simulink model "LQG"  (R2019a)
settings: Solver=VariableStepAuto  StartTime=0.0  StopTime=50  RelTol=1e-3  EnableMultiTasking=on
values from neighbouring files (symbols this model uses):
  C = [1 0 0 0 0 0]    [FinalProjectENPM667.m]
  K = lqr(A, B, Q, R)    [FinalProjectENPM667.m]
  l1 = 20    [FinalProjectENPM667.m]
  l2 = 10    [FinalProjectENPM667.m]
  M = 1000    [FinalProjectENPM667.m]
  m1 = 100    [FinalProjectENPM667.m]
  m2 = 100    [FinalProjectENPM667.m]
undefined symbols (not defined in the file or in its folder): A1, B1, Continuous, Nbar, Time, X0
libraries: ctrlSharedLib x1
settings Model: Creator=Rishabh  LastModifiedBy=detwieller
settings DataIOCC: ReturnWorkspaceOutputs=off
settings OptimizationCC: LifeSpan=inf
settings DebuggingCC: SFUnexpectedBacktrackingDiag=warning  SFNoUnconditionalDefaultTransitionDiag=warning  SFExecutionAtInitializationDiag=none  ArithmeticOperatorsInVariantConditions=warning
settings SFSimCC: SimUseLocalCustomCode=off
settings RTWCC: RTWUseLocalCustomCode=off
settings CodeAppCC: StateflowObjectComments=on
settings GRTTargetCC: TargetLangStandard=C89/C90 (ANSI)  GeneratePreprocessorConditionals=Disable all
settings ConfigComp: CovMetricSettings=dw  CovHtmlReporting=on  CovSaveCumulativeToWorkspaceVar=on  CovSaveSingleToWorkspaceVar=on  CovExternalEMLEnable=off

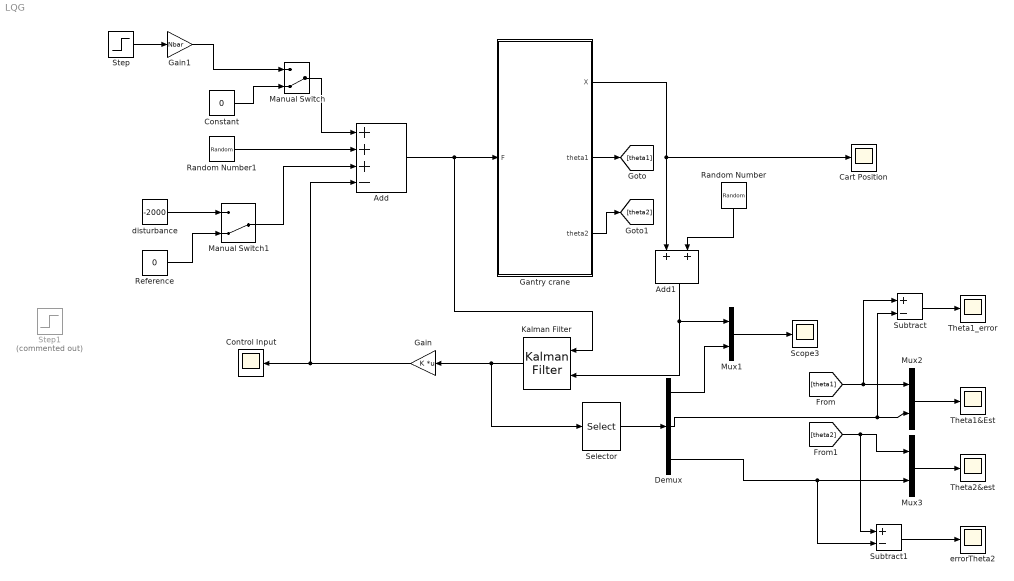
== system LQG ==
  Add : Sum  Inputs=+++-
  Add1 : Sum
  Cart Position : Scope
  Constant : Constant  Value=0
  Control Input : Scope
  Demux : Demux  Outputs=3
  Gain : Gain  Gain=K  Multiplication=Matrix(K*u)
  Gain1 : Gain  Gain=Nbar
  "Gantry crane " : Subsystem
  Kalman Filter : ctrlSharedLib/Kalman Filter  TimeDomain=Continuous-Time  UseCurrentEstimator=on  ModelSource=Individual A, B, C, D matrices  ModelSourceVariable=ss(0.95,1,1,0,1)  A=A1  B=B1  C=C  D=0  NumberOfStates=1  NumberOfInputs=1  NumberOfOutputs=1  InitialEstimateSource=Dialog  X0=[0 0 X0(3) 0 X0(5) 0]  P0=10  UseK=off  UseGH=on  NumberOfProcessNoiseInputs=1  G=B1  TimeInvariantG=on  H=0  TimeInvariantH=on  Q=0.2  TimeInvariantQ=on  R=0.001  TimeInvariantR=on  N=0  TimeInvariantN=on  AddInputPort=on  AddEnablePort=off  OutputEstimatedY=off  OutputP=off  Ts=-1
      settings: SourceProductBaseCode=CT
  Manual Switch : ManualSwitch  CurrentSetting=0
  Manual Switch1 : ManualSwitch  CurrentSetting=0
  Mux1 : Mux  Inputs=2
  Mux2 : Mux  Inputs=2
  Mux3 : Mux  Inputs=2
  Random Number : RandomNumber  Variance=0.001  SampleTime=0.1
  Random Number1 : RandomNumber  Variance=0.2  SampleTime=0.1
  Reference : Constant  Value=0
  Scope3 : Scope
  Selector : Selector  InputPortWidth=6  IndexOptions=Index vector (dialog)  Indices=[1 3 5]  OutputSizes=1
  Step : Step  After=10  SampleTime=0
  Step1 : Step  Commented=on  After=500  SampleTime=0
  Subtract : Sum  Inputs=+-
  Subtract1 : Sum  Inputs=+-
  Theta1&Est : Scope
  Theta1_error : Scope
  Theta2&est : Scope
  disturbance : Constant  Value=-2000
  "errorTheta2 " : Scope
  wires:
  "Gantry crane "/1(X) -> Add1/1, Cart Position/1
  Add1/1 -> Mux1/1, Kalman Filter/2
  Kalman Filter/1 -> Gain/1, Selector/1
  Mux1/1 -> Scope3/1
  [theta1] -> Subtract/1, Mux2/1
  [theta2] -> Subtract1/1, Mux3/1
  Mux2/1 -> Theta1&Est/1
  Mux3/1 -> Theta2&est/1
  "Gantry crane "/2(theta1) -> [theta1]
  "Gantry crane "/3(theta2) -> [theta2]
  Subtract/1 -> Theta1_error/1
  Subtract1/1 -> "errorTheta2 "/1
  Constant/1 -> Manual Switch/2
  Manual Switch/1 -> Add/1
  Random Number/1 -> Add1/2
  Random Number1/1 -> Add/2
  Gain/1 -> Control Input/1, Add/4
  Step/1 -> Gain1/1
  Gain1/1 -> Manual Switch/1
  Add/1 -> Kalman Filter/1, "Gantry crane "/1(F)
  disturbance/1 -> Manual Switch1/1
  Reference/1 -> Manual Switch1/2
  Manual Switch1/1 -> Add/3
  Selector/1 -> Demux/1
  Demux/1 -> Mux1/2
  Demux/2 -> Subtract/2, Mux2/2
  Demux/3 -> Subtract1/2, Mux3/2

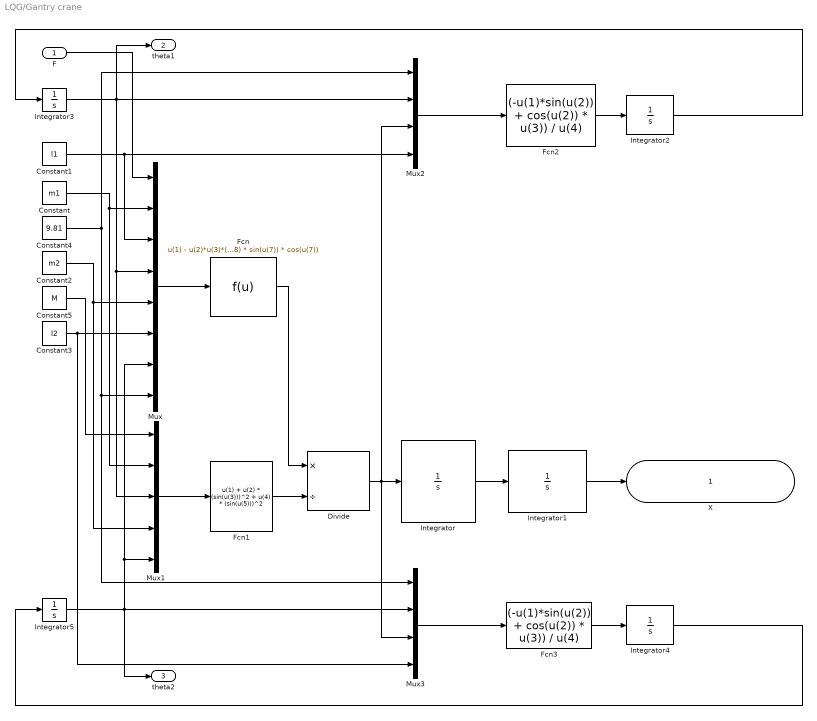
== system LQG/Gantry crane  ==
  F : Inport
  Constant : Constant  Value=m1
  Constant1 : Constant  Value=l1
  Constant2 : Constant  Value=m2
  Constant3 : Constant  Value=l2
  Constant4 : Constant  Value=9.81
  Constant5 : Constant  Value=M
  Divide : Product  Inputs=*/
  Fcn : Fcn  Expr=u(1) - u(2)*u(3)*(u(4)^2)*sin(u(4)) - u(5) * u(6) * (u(7)^2)*sin(u(7))-u(2)*u(8)*sin(u(4))*cos(u(4)) - u(5) * u(8) * sin(u(7)) * cos(u(7))
  Fcn1 : Fcn  Expr=u(1) + u(2) * (sin(u(3)))^2 + u(4) * (sin(u(5)))^2
  Fcn2 : Fcn  Expr=(-u(1)*sin(u(2)) + cos(u(2)) * u(3)) / u(4)
  Fcn3 : Fcn  Expr=(-u(1)*sin(u(2)) + cos(u(2)) * u(3)) / u(4)
  Integrator : Integrator
  Integrator1 : Integrator  InitialCondition=X0(1)
  Integrator2 : Integrator
  Integrator3 : Integrator  InitialCondition=X0(3)
  Integrator4 : Integrator
  Integrator5 : Integrator  InitialCondition=X0(5)
  Mux : Mux  Inputs=8
  Mux1 : Mux  Inputs=5
  Mux2 : Mux
  Mux3 : Mux
  X : Outport
  theta1 : Outport  Port=2
  theta2 : Outport  Port=3
  wires:
  Integrator5/1 -> Mux/7, Mux1/5, Mux3/2, theta2/1
  Divide/1 -> Mux3/3, Mux2/3, Integrator/1
  Constant/1 -> Mux1/2, Mux/2
  Constant1/1 -> Mux2/4, Mux/3
  Mux/1 -> Fcn/1
  Integrator3/1 -> Mux1/3, Mux/4, Mux2/2, theta1/1
  Fcn/1 -> Divide/1
  F/1 -> Mux/1
  Integrator1/1 -> X/1
  Integrator2/1 -> Integrator3/1
  Fcn2/1 -> Integrator2/1
  Mux3/1 -> Fcn3/1
  Fcn3/1 -> Integrator4/1
  Constant3/1 -> Mux3/4, Mux/6
  Fcn1/1 -> Divide/2
  Constant2/1 -> Mux1/4, Mux/5
  Mux2/1 -> Fcn2/1
  Mux1/1 -> Fcn1/1
  Integrator/1 -> Integrator1/1
  Constant4/1 -> Mux3/1, Mux/8, Mux2/1
  Constant5/1 -> Mux1/1
  Integrator4/1 -> Integrator5/1
